simulink library "dspxfrm2"  (Simulink 3.00)
undefined symbols (not defined in the file or in its folder): magnitude
libraries: dspxfrm2 x4, dspbdsp2 x2, dspvect2 x1
settings Model: RequirementInfo=9  Creator=szlotkin  LastModifiedBy=jeff

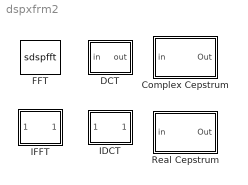
== system dspxfrm2 ==
  Complex Cepstrum : Subsystem  mask(Complex Cepstrum){N=64}
      mask prompts: N "FFT length:"
      mask help: Complex cepstrum of input signal. Input is modified to remove possible phase discontinuity at +/- pi radians.
      mask init:
      | if isempty(N),
      |  nh=1; lag=1;
      | else
      |   nh = fix((N+1)/2); lag = pi*(0:(N-1))/nh;
      | end
      mask Help: web(dspbhelp);
      mask Display: disp('Complex\n Cepstrum')
  DCT : Subsystem  mask(DCT){nChans=1}
      mask prompts: nChans "Number of channels:"
      mask help: Discrete cosine transform of a real or complex input vector. Input frame size must be a power of 2.
      mask Help: web(dspbhelp);
      mask Display: disp(' DCT')
  FFT : S-Function  FunctionName=sdspfft  Parameters=nchans  PortCounts=[]  mask(FFT){nchans=1}
      mask prompts: nchans "Number of channels:"
      mask help: Fast Fourier transform with complex output. Input frame size must be a power of 2.
      mask Help: web(dspbhelp);
      mask Display: disp('  FFT ');
  IDCT : Subsystem  mask(IDCT){nchans=1}
      mask prompts: nchans "Number of channels:"
      mask help: Inverse discrete cosine transform of a real vector. Input frame size must be a power of 2.
      mask Help: web(dspbhelp);
      mask Display: disp('IDCT')
  IFFT : Subsystem  mask(IFFT){mode=Real, cs_in=off, nchans=1}
      mask prompts: mode "Output:"; cs_in "Conjugate symmetric input"; nchans "Number of channels:"
      mask help: Inverse fast Fourier transform of a complex input vector with real or complex output. Input frame size must be a power of 2.
      mask init:
      | realmode = (mode == 1);
      | if ( cs_in == 1), mode = 3; end;
      mask Help: web(dspbhelp);
      mask StyleString: popup(Real|Complex),checkbox,edit
      mask CallbackString: dspblkifft||
      mask Display: disp('  IFFT')
  Real Cepstrum : Subsystem  mask(Real Cepstrum){N=64}
      mask prompts: N "FFT length:"
      mask help: Real cepstrum of input signal.
      mask Help: web(dspbhelp);
      mask Display: disp('Real\nCepstrum')

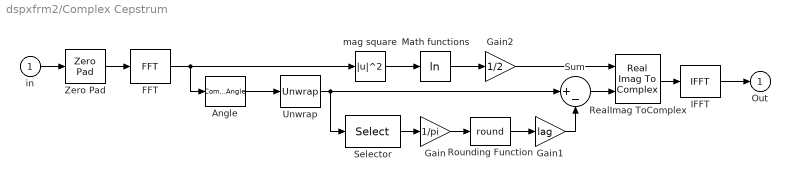
== system dspxfrm2/Complex Cepstrum ==
  in : Inport  Port=1
  Angle : ComplexToMagnitudeAngle  Output=Angle
  FFT : dspxfrm2/FFT  nchans=1
  Gain : Gain  Gain=1/pi  Multiplication=Element-wise(K.*u)  SaturateOnIntegerOverflow=on
  Gain1 : Gain  Gain=lag  Multiplication=Element-wise(K.*u)  SaturateOnIntegerOverflow=on
  Gain2 : Gain  Gain=1/2  Multiplication=Element-wise(K.*u)  SaturateOnIntegerOverflow=on
  IFFT : dspxfrm2/IFFT  mode=Real  cs_in=off  nchans=1
  Math functions : Math  Operator=log  OutputSignalType=auto
  RealImag ToComplex : RealImagToComplex  Input=RealAndImag  ConstantPart=0
  Rounding Function : Rounding  Operator=round
  Selector : Selector  Elements=nh+1  InputPortWidth=N
  Sum : Sum  Inputs=|+-  SaturateOnIntegerOverflow=on
  Unwrap : dspvect2/Unwrap  tol=pi
  Zero Pad : dspbdsp2/Zero Pad  pad=N  trunc=on  nchans=1
  mag square : Math  Operator=magnitude^2  OutputSignalType=auto
  Out : Outport  Port=1  InitialOutput=0
  wires:
  mag square/1 -> Math functions/1
  Math functions/1 -> Gain2/1
  in/1 -> Zero Pad/1
  Zero Pad/1 -> FFT/1
  FFT/1 -> Angle/1, mag square/1
  Rounding Function/1 -> Gain1/1
  Gain/1 -> Rounding Function/1
  Selector/1 -> Gain/1
  Unwrap/1 -> Sum/1, Selector/1
  Angle/1 -> Unwrap/1
  Gain1/1 -> Sum/2
  RealImag ToComplex/1 -> IFFT/1
  Sum/1 -> RealImag ToComplex/2
  Gain2/1 -> RealImag ToComplex/1
  IFFT/1 -> Out/1

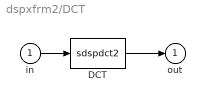
== system dspxfrm2/DCT ==
  in : Inport  Port=1
  DCT : S-Function  FunctionName=sdspdct2  Parameters=nChans  PortCounts=[]
  out : Outport  Port=1  InitialOutput=0
  wires:
  in/1 -> DCT/1
  DCT/1 -> out/1

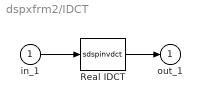
== system dspxfrm2/IDCT ==
  in_1 : Inport  Port=1
  Real IDCT : S-Function  FunctionName=sdspinvdct  Parameters=nchans  PortCounts=[]
  out_1 : Outport  Port=1  InitialOutput=0
  wires:
  in_1/1 -> Real IDCT/1
  Real IDCT/1 -> out_1/1

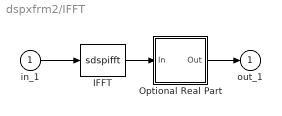
== system dspxfrm2/IFFT ==
  in_1 : Inport  Port=1
  IFFT : S-Function  FunctionName=sdspifft  Parameters=mode,nchans  PortCounts=[]
  Optional Real Part : Subsystem  mask(Replaceable Contents){oname=Real, osrc=built-in/ComplexToRealImag, oargs={'output','Real'}, replace=~realmode}
      mask prompts: oname "Relative name of blocks to replace:"; osrc "Simulink path to each source block:"; oargs "Parameter/value pairs to each block:"; replace "Replace with short-circuit:"
      mask help: Configurable subsystem holding blocks which may be replaced by virtual short-circuits (muxes) when not needed.
      mask init:
      | opts.name = oname; opts.src = osrc; opts.args = oargs;
      | dspskipblk(gcb,opts,replace);
  out_1 : Outport  Port=1  InitialOutput=0
  wires:
  in_1/1 -> IFFT/1
  IFFT/1 -> Optional Real Part/1(In)
  Optional Real Part/1(Out) -> out_1/1

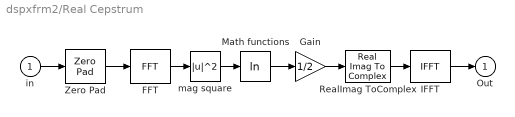
== system dspxfrm2/Real Cepstrum ==
  in : Inport  Port=1
  FFT : dspxfrm2/FFT  nchans=1
  Gain : Gain  Gain=1/2  Multiplication=Element-wise(K.*u)  SaturateOnIntegerOverflow=on
  IFFT : dspxfrm2/IFFT  mode=Real  cs_in=off  nchans=1
  Math functions : Math  Operator=log  OutputSignalType=auto
  RealImag ToComplex : RealImagToComplex  Input=Real  ConstantPart=0
  Zero Pad : dspbdsp2/Zero Pad  pad=N  trunc=on  nchans=1
  mag square : Math  Operator=magnitude^2  OutputSignalType=auto
  Out : Outport  Port=1  InitialOutput=0
  wires:
  Zero Pad/1 -> FFT/1
  in/1 -> Zero Pad/1
  FFT/1 -> mag square/1
  mag square/1 -> Math functions/1
  Math functions/1 -> Gain/1
  Gain/1 -> RealImag ToComplex/1
  RealImag ToComplex/1 -> IFFT/1
  IFFT/1 -> Out/1

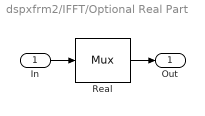
== system dspxfrm2/IFFT/Optional Real Part ==
  In : Inport  Port=1
  Real : Mux  Inputs=1
      settings: DisplayOption=none
  Out : Outport  Port=1  InitialOutput=0
  wires:
  In/1 -> Real/1
  Real/1 -> Out/1
